simulink model "openlooptest"  (R2023a)
settings: Solver=VariableStepAuto  StartTime=0.0  StopTime=21  RelTol=1e-3
values from neighbouring files (symbols this model uses):
  g = 9.81    [steady_state_torques.m]
  I_noload = 0.26    [MotorParameters.m]
  K_m = 27e-3    (= 0.027)    [MotorParameters.m]
  l = 0.1    [steady_state_torques.m]
  m = 0.1    [steady_state_torques.m]
  R = 2    [MotorParameters.m]
undefined symbols (not defined in the file or in its folder): init, wave_amplitude, wave_offset, wave_period
settings Model: Creator=yunzh  LastModifiedBy=yunzh

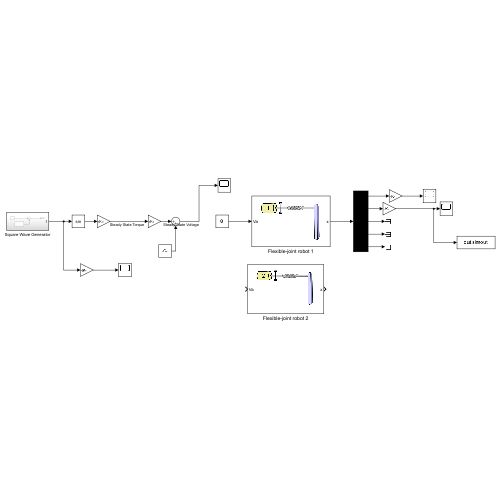
[thumbnail: Simulink's stored preview of the top-level diagram]
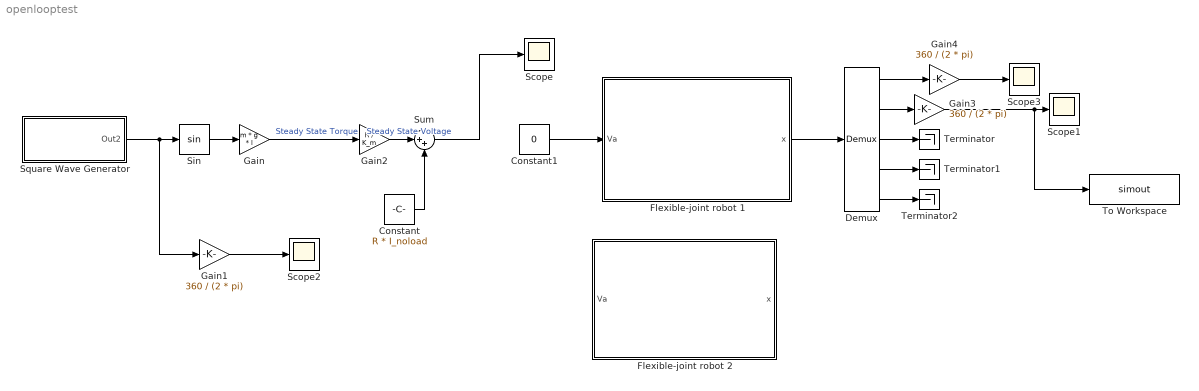
== system openlooptest ==
  Constant : Constant  Value=R * I_noload
  Constant1 : Constant  Value=0
  Demux : Demux  Outputs=5
  Flexible-joint robot 1 : Subsystem
      mask Display: image('$imagefile'); % Use "Edit Image" on toolstrip to change.
  Flexible-joint robot 2 : Subsystem
      mask Display: image('$imagefile'); % Use "Edit Image" on toolstrip to change.
  Gain : Gain  Gain=m * g * l
  Gain1 : Gain  Gain=360 / (2 * pi)
  Gain2 : Gain  Gain=R / K_m
  Gain3 : Gain  Gain=360 / (2 * pi)
  Gain4 : Gain  Gain=360 / (2 * pi)
  Scope{,1..3} (4 alike) : Scope
  Sin : Trigonometry
  Square Wave Generator : Subsystem
  Sum : Sum  Inputs=|++
  Terminator : Terminator
  Terminator1 : Terminator
  Terminator2 : Terminator
  To Workspace : ToWorkspace  VariableName=simout  SaveFormat=Timeseries  SampleTime=-1
  wires:
  Square Wave Generator/1(Out2) -> Sin/1, Gain1/1
  Gain1/1 -> Scope2/1
  Sin/1 -> Gain/1
  Gain/1 -> Gain2/1  "Steady State Torque"
  Demux/2 -> Gain3/1
  Demux/3 -> Terminator/1
  Demux/1 -> Gain4/1
  Demux/4 -> Terminator1/1
  Demux/5 -> Terminator2/1
  Gain3/1 -> To Workspace/1, Scope1/1
  Gain2/1 -> Sum/1  "Steady State Voltage"
  Sum/1 -> Scope/1
  Constant/1 -> Sum/2
  Gain4/1 -> Scope3/1
  Flexible-joint robot 1/1(x) -> Demux/1
  Constant1/1 -> Flexible-joint robot 1/1(Va)

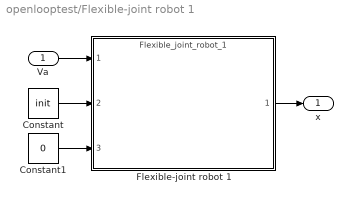
== system openlooptest/Flexible-joint robot 1 ==
  Va : Inport
  Constant : Constant  Value=init
  Constant1 : Constant  Value=0
  Flexible-joint robot 1 : ModelReference  ModelNameDialog=Flexible_joint_robot_1  ModelReferenceVersion=1.65  CopyOfModelProtected=on
  x : Outport
  wires:
  Constant/1 -> Flexible-joint robot 1/2
  Constant1/1 -> Flexible-joint robot 1/3
  Flexible-joint robot 1/1 -> x/1
  Va/1 -> Flexible-joint robot 1/1

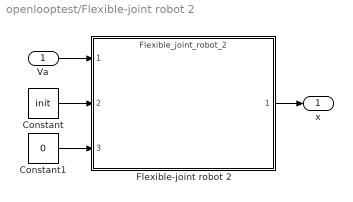
== system openlooptest/Flexible-joint robot 2 ==
  Va : Inport
  Constant : Constant  Value=init
  Constant1 : Constant  Value=0
  Flexible-joint robot 2 : ModelReference  ModelNameDialog=Flexible_joint_robot_2  ModelReferenceVersion=1.65  CopyOfModelProtected=on
  x : Outport
  wires:
  Va/1 -> Flexible-joint robot 2/1
  Constant1/1 -> Flexible-joint robot 2/3
  Constant/1 -> Flexible-joint robot 2/2
  Flexible-joint robot 2/1 -> x/1

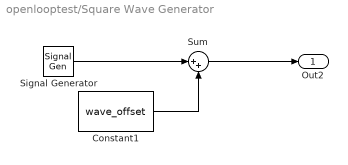
== system openlooptest/Square Wave Generator ==
  Constant1 : Constant  Value=wave_offset
  Signal Generator : SignalGenerator  WaveForm=square  Amplitude=wave_amplitude  Frequency=1 / wave_period
  Sum : Sum  Inputs=|++
  Out2 : Outport
  wires:
  Signal Generator/1 -> Sum/1
  Constant1/1 -> Sum/2
  Sum/1 -> Out2/1
